simulink model "Lab3"  (R2018a)
settings: Solver=VariableStepAuto  StartTime=0.0  StopTime=Time  RelTol=1e-3
values from neighbouring files (symbols this model uses):
  cp = 0.8    [Workspace.m]
  cs = 0.05    [Workspace.m]
  dd = 1.15    [Workspace.m]
  dp = 0    [Workspace.m]
  hd = 1.3    [Workspace.m]
  hi = 0    [Workspace.m]
  hp = 0    [Workspace.m]
  kp = 6.32    [Workspace.m]
  ks = 0.0632    [Workspace.m]
  mp = 0.16    [Workspace.m]
  ms = 0.16    [Workspace.m]
  sinefreq = w/2    [Workspace.m]
  T = 0.1450    (= 0.145)    [Workspace.m]
  w = sinefreq/2    [Workspace.m]
  z = cp/(2*sqrt(kp*mp))    [Workspace.m]
settings Model: Creator=c_s  LastModifiedBy=c_s

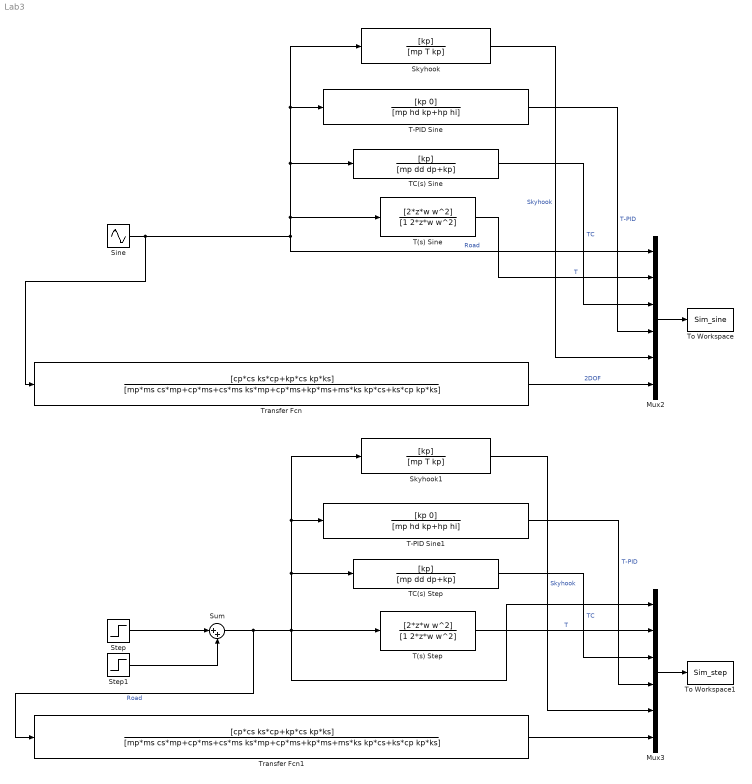
== system Lab3 ==
  Mux2 : Mux  Inputs=6
  Mux3 : Mux  Inputs=6
  Sine : Sin  Amplitude=0.05  Frequency=sinefreq  SampleTime=0
  Skyhook : TransferFcn  Numerator=[kp]  Denominator=[mp T kp]
  Skyhook1 : TransferFcn  Numerator=[kp]  Denominator=[mp T kp]
  Step : Step  After=0.05  SampleTime=0
  Step1 : Step  Time=2  After=-0.05  SampleTime=0
  Sum : Sum  Inputs=|++
  T(s) Sine : TransferFcn  Numerator=[2*z*w w^2]  Denominator=[1 2*z*w w^2]
  T(s) Step : TransferFcn  Numerator=[2*z*w w^2]  Denominator=[1 2*z*w w^2]
  T-PID Sine : TransferFcn  Numerator=[kp 0]  Denominator=[mp hd kp+hp hi]
  T-PID Sine1 : TransferFcn  Numerator=[kp 0]  Denominator=[mp hd kp+hp hi]
  TC(s) Sine : TransferFcn  Numerator=[kp]  Denominator=[mp dd dp+kp]
  TC(s) Step : TransferFcn  Numerator=[kp]  Denominator=[mp dd dp+kp]
  To Workspace : ToWorkspace  VariableName=Sim_sine  SaveFormat=Structure With Time  SampleTime=-1
  To Workspace1 : ToWorkspace  VariableName=Sim_step  SaveFormat=Structure With Time  SampleTime=-1
  Transfer Fcn : TransferFcn  Numerator=[cp*cs ks*cp+kp*cs kp*ks]  Denominator=[mp*ms cs*mp+cp*ms+cs*ms ks*mp+cp*ms+kp*ms+ms*ks kp*cs+ks*cp kp*ks]
  Transfer Fcn1 : TransferFcn  Numerator=[cp*cs ks*cp+kp*cs kp*ks]  Denominator=[mp*ms cs*mp+cp*ms+cs*ms ks*mp+cp*ms+kp*ms+ms*ks kp*cs+ks*cp kp*ks]
  wires:
  T(s) Sine/1 -> Mux2/2  "T"
  Sine/1 -> Transfer Fcn/1, TC(s) Sine/1, Skyhook/1, T-PID Sine/1, T(s) Sine/1, Mux2/1  "Road"
  Mux2/1 -> To Workspace/1
  Step/1 -> Sum/1
  Step1/1 -> Sum/2
  TC(s) Sine/1 -> Mux2/3  "TC"
  Mux3/1 -> To Workspace1/1
  Sum/1 -> Transfer Fcn1/1, Skyhook1/1, T-PID Sine1/1, TC(s) Step/1, Mux3/1, T(s) Step/1  "Road"
  T(s) Step/1 -> Mux3/2  "T"
  TC(s) Step/1 -> Mux3/3  "TC"
  T-PID Sine1/1 -> Mux3/4  "T-PID"
  T-PID Sine/1 -> Mux2/4  "T-PID"
  Skyhook/1 -> Mux2/5  "Skyhook"
  Skyhook1/1 -> Mux3/5  "Skyhook"
  Transfer Fcn/1 -> Mux2/6  "2DOF"
  Transfer Fcn1/1 -> Mux3/6
